simulink model "stewart_platform_tests"  (R2019b)
settings: configuration reference "conf_simscape" (kept outside this file)
libraries: sm_lib x2, nesl_utility x1
settings Model: Creator=thomas  LastModifiedBy=thomas
settings ConfigSetRef: SourceName=conf_simscape  SourceLocation=Base Workspace

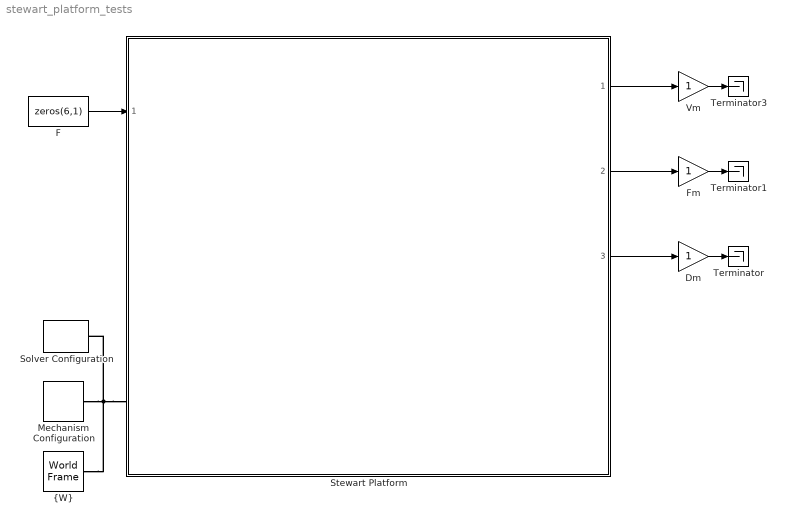
== system stewart_platform_tests ==
  Dm : Gain
  F : Constant  Value=zeros(6,1)
  Fm : Gain
  Mechanism Configuration : sm_lib/Utilities/Mechanism Configuration  UniformGravity=None  GravityVector=[0 0 0]  GravityUnits=m/s^2  LinearizationDelta=0.001
  Solver Configuration : nesl_utility/Solver Configuration  PhysicalDomain=network_engine_domain  SubClassName=solver  LeftPortType=input  RightPortType=generic  Tones=[]  Harmonics=[]  SimulateNoise=off  Profile=off  UseLocalSampling=off  EnableSwitchedLinearOptims=on  FrequencyDomain=off  UseCCode=off  RelTol=0.001  AbsTol=1e-06  MinStep=1e-09  ToWorkspace=off  RevertToSquareIcSolve=off  NumHomotopyIterations=100  PhasorMode=off  PhasorModeNumHarmonics=1  DoDC=off  ResidualTolerance=1e-09  UseLocalSolver=off  LocalSolverChoice=NE_BACKWARD_EULER_ADVANCER  LocalSolverSampleTime=0.001  DoFixedCost=off  MaxNonlinIter=3  MaxModeIter=2  LinearAlgebra=auto  EquationFormulation=NE_TIME_EF  DelaysMemoryBudget=1024  AutomaticFiltering=on  FilteringTimeConstant=0.001  PartitionStorageMethod=AS_NEEDED  PartitionMemoryBudget=1024  PartitionMethod=ROBUST
  Stewart Platform : Subsystem  ReferencedSubsystem=Stewart_Platform
  Terminator : Terminator
  Terminator1 : Terminator
  Terminator3 : Terminator
  Vm : Gain
  "{W}" : sm_lib/Frames and Transforms/World Frame
  wires:
  Vm/1 -> Terminator3/1
  Stewart Platform/3 -> Dm/1
  Fm/1 -> Terminator1/1
  Stewart Platform/1 -> Vm/1
  F/1 -> Stewart Platform/1
  Stewart Platform/2 -> Fm/1
  Dm/1 -> Terminator/1
  connections:
  Mechanism Configuration/RConn1 -- Solver Configuration/RConn1 -- Stewart Platform/LConn2 -- "{W}"/RConn1
